simulink model "Stepdown Bridge Cycloconverter"  (R2017a)
settings: Solver=ode23tb  StartTime=0.0  StopTime=0.2  MaxStep=0.001  RelTol=1e-3  EnableMultiTasking=on
libraries: powerlib x16
settings Model: Creator=uwss  LastModifiedBy=sujee
settings DataIOCC: LimitDataPoints=on  SaveFormat=Array  SignalLoggingSaveFormat=ModelDataLogs
settings OptimizationCC: ExpressionDepthLimit=2147483647  LifeSpan=inf
settings DebuggingCC: UnderspecifiedInitializationDetection=Classic  MergeDetectMultiDrivingBlocksExec=none  SolverPrmCheckMsg=warning  FcnCallInpInsideContextMsg=warning  StateNameClashWarn=warning  SFUnexpectedBacktrackingDiag=warning  SFNoUnconditionalDefaultTransitionDiag=warning  SFExecutionAtInitializationDiag=none
settings HardwareCC: ProdBitPerPointer=32  ProdBitPerSizeT=32  ProdBitPerPtrDiffT=32  ProdLargestAtomicFloat=None  ProdIntDivRoundTo=Undefined  ProdEndianess=Unspecified  ProdWordSize=32  ProdHWDeviceType=32-bit Generic
settings ModelReferenceCC: PropagateSignalLabelsOutOfModel=off
settings GRTTargetCC: TargetLangStandard=C89/C90 (ANSI)  CombineOutputUpdateFcns=off  GRTInterface=on
settings ConfigComp: CovMetricSettings=dw  CovSaveCumulativeToWorkspaceVar=on  CovSaveSingleToWorkspaceVar=on

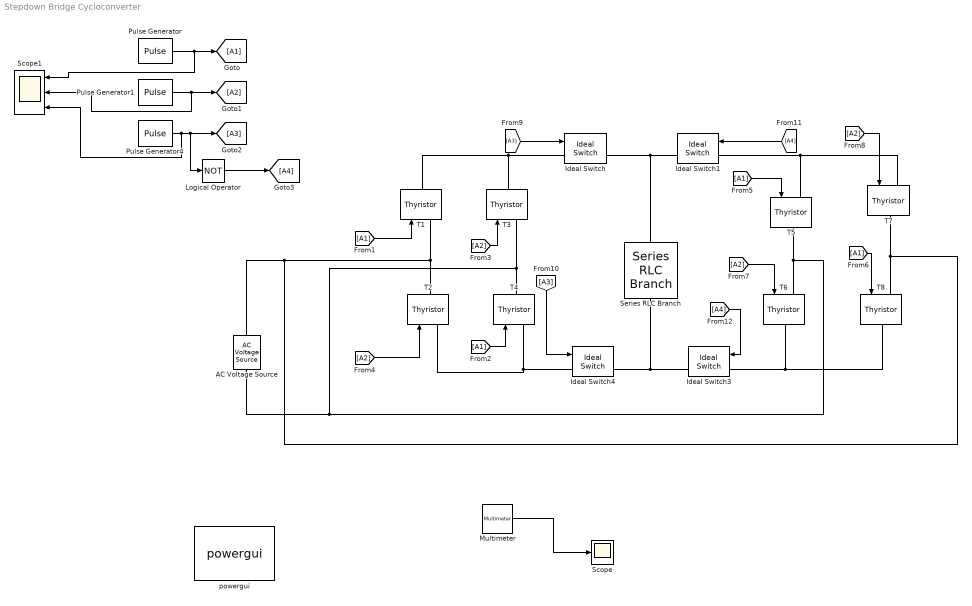
== system Stepdown Bridge Cycloconverter ==
  AC Voltage Source : powerlib/Electrical Sources/AC Voltage Source  Amplitude=100  Phase=0  Frequency=50  SampleTime=0  Measurements=None  BusType=swing  Pref=10e3  Qref=0  Qmin=-inf  Qmax=+inf
  Ideal Switch{,1,3..4} (4 alike) : powerlib/Power Electronics/Ideal Switch  Ron=0.001  Lon=0  IC=0  Rs=1e5  Cs=inf  Measurements=on
  Logical Operator : Logic  Operator=NOT  AllPortsSameDT=off  OutDataTypeStr=boolean
  Multimeter : powerlib/Measurements/Multimeter  PhasorSimulation=off  OutputType=Complex  sel=1  L=1  Gain=1  yselected={'Ub: Series RLC Branch'};  PSBOutputType=1  PSBequivalent=0  AxesSetting=[0,0.1,-100,100]  Display=1  SavedBlockNames=-11
  Pulse Generator : DiscretePulseGenerator  PulseType=Time based  Period=0.002  PulseWidth=5
  Pulse Generator1 : DiscretePulseGenerator  PulseType=Time based  Period=0.002  PulseWidth=5  PhaseDelay=(0.002/360)*180
  Pulse Generator4 : DiscretePulseGenerator  PulseType=Time based  Period=0.194  PulseWidth=50
  Scope : Scope
  Scope1 : Scope  NumInputPorts=3
  Series RLC Branch : powerlib/Elements/Series RLC Branch  LConnTagsString=__new0  RConnTagsString=__new0  BranchType=R  Resistance=10  Inductance=1e-3  SetiL0=off  InitialCurrent=0  Capacitance=1.0  Setx0=off  InitialVoltage=0  Measurements=Branch voltage
  T{1..4} (4 alike) : powerlib/Power Electronics/Thyristor  Ron=0.001  Lon=0  Vf=0.8  IC=0  Rs=5000  Cs=250e-9  Measurements=off
  T{5..8} (4 alike) : powerlib/Power Electronics/Thyristor  Ron=0.001  Lon=0  Vf=0.8  IC=0  Rs=500  Cs=250e-9  Measurements=off
  powergui : powerlib/powergui  Priority=1  SimulationMode=Discrete  SampleTime=50e-6  frequency=60  Iterations=50  frequencyindice=50  Pbase=100e6  ErrMax=1e-4  UnitsV=kV  UnitsW=MW  buscounter=0  FunctionMessages=off  echomessages=off  EnableUseOfTLC=off  CurrentSourceSwitches=off  DisableSnubberDevices=off  DisableRonSwitches=off  DisableVfSwitches=off  DisplayEquations=off  AutomaticDiscreteSolvers=off  SolverType=Tustin/Backward Euler (TBE)  Interpol=off  ExternalGateDelay=off  methode=off  Ts=0  x0status=blocks  SPID=off  SwTol=0  HookPort=off  NonlinearTolerance=1e-4  nMaxIteration=100  ContinueOnMaxIteration=off  RestoreLinks=warning  ResistiveCurrentMeasurement=off  Frange=[0:2:500]  Ylog=off  Xlog=on  ShowGrid=off  save=off  variable=ZData  structure=cycloconverter  ZoomFFT=off  StartTime=0.4  cycles=1  DisplayStyle=4  fundamental=5  FreqAxis=off  MaxFrequency=1000  frequencyindicesteady=1  RmsSteady=1  display=off
  wires:
  Pulse Generator4/1 -> Scope1/3, [A3], Logical Operator/1
  Pulse Generator/1 -> Scope1/1, [A1]
  [A1] -> T1/1
  [A1] -> T4/1
  [A2] -> T2/1
  [A2] -> T3/1
  Pulse Generator1/1 -> Scope1/2, [A2]
  [A1] -> T8/1
  [A2] -> T7/1
  [A2] -> T6/1
  [A3] -> Ideal Switch4/1
  Logical Operator/1 -> [A4]
  [A4] -> Ideal Switch1/1
  [A4] -> Ideal Switch3/1
  [A3] -> Ideal Switch/1
  [A1] -> T5/1
  Multimeter/1 -> Scope/1
  connections:
  AC Voltage Source/RConn1 -- T1/LConn1 -- T2/RConn1 -- T7/RConn1 -- T8/LConn1
  T6/LConn1 -- AC Voltage Source/LConn1 -- T3/LConn1 -- T4/RConn1 -- T5/RConn1
  Ideal Switch4/RConn1 -- Series RLC Branch/RConn1 -- Ideal Switch3/RConn1
  Ideal Switch/LConn1 -- T3/RConn1 -- T1/RConn1
  T7/LConn1 -- T5/LConn1 -- Ideal Switch1/LConn1
  Series RLC Branch/LConn1 -- Ideal Switch/RConn1 -- Ideal Switch1/RConn1
  T8/RConn1 -- T6/RConn1 -- Ideal Switch3/LConn1
  T4/LConn1 -- T2/LConn1 -- Ideal Switch4/LConn1
